simulink model "LQI_NL_simulation"  (R2024b)
settings: Solver=VariableStepAuto  StartTime=0.0  StopTime=20  RelTol=1e-3
values from neighbouring files (symbols this model uses):
  A_kf = A_ext - L_kf*C_meas    [SS_model_LQ.m]
  B_kf = [L_kf B_ext]    [SS_model_LQ.m]
  C_kf = eye(3)    [SS_model_LQ.m]
  D_kf = zeros(3,3)    [SS_model_LQ.m]
  g = 9.81    [LQI_Giuse_code.m]    (also in SS_model_LQ.m)
  G_i_num = G_i_num(2)    [SS_model_LQ.m]
  i_e = sqrt((m*g/km) * (x_e + 2*r -l)^2)    [SS_model_LQ.m]
  K_aug = lqr(A_aug, B_aug, Q_aug, R_aug)    [SS_model_LQ.m]
  Kg = 3    [LQI_Giuse_code.m]    (also in SS_model_LQ.m)
  Ki_i = Ki_p/Ti    [LQI_Giuse_code.m]    (also in SS_model_LQ.m = 1650.02619)
  km = 6.5308e-5    (= 6.5308e-05)    [LQI_Giuse_code.m]    (also in SS_model_LQ.m)
  Kp_i = 72.795273    [SS_model_LQ.m]
  l = 0.0394    [LQI_Giuse_code.m]    (also in SS_model_LQ.m)
  L = 412.5e-3    (= 0.4125)    [SS_model_LQ.m]
  m = 0.068    [LQI_Giuse_code.m]    (also in SS_model_LQ.m)
  r = 1.27e-2    (= 0.0127)    [LQI_Giuse_code.m]    (also in SS_model_LQ.m)
  R = 1    [LQI_Giuse_code.m]    (also in SS_model_LQ.m = 9.35)
  x_e = [x1_e, x2_e]    [LQI_Giuse_code.m]    (also in SS_model_LQ.m = 0.007)
undefined symbols (not defined in the file or in its folder): G_i_den
libraries: slpidlib x1
settings Model: Creator=edoardo  LastModifiedBy=edoardo

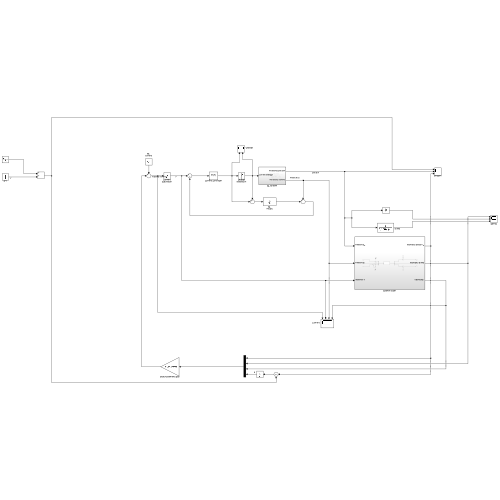
[thumbnail: Simulink's stored preview of the top-level diagram]
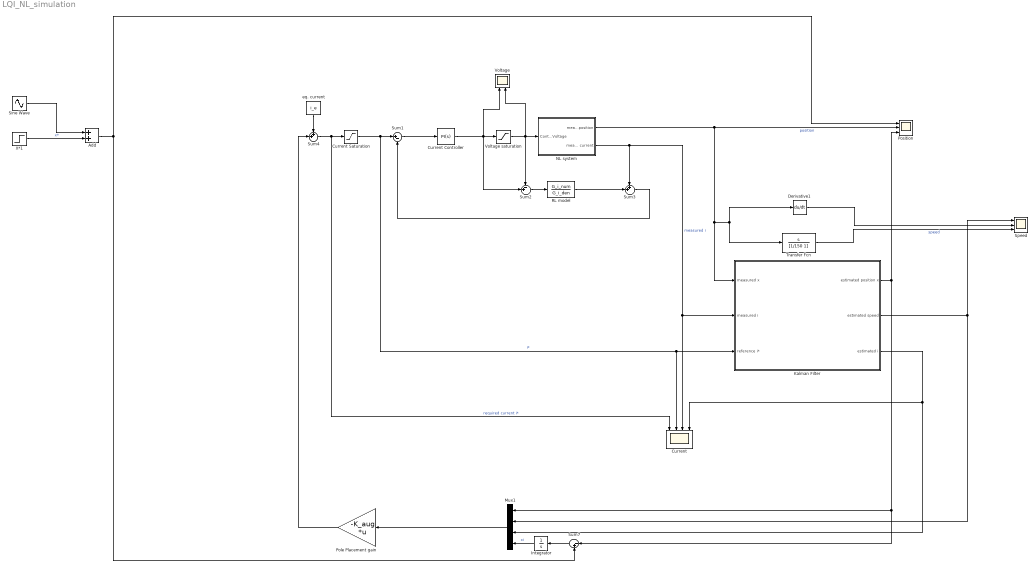
== system LQI_NL_simulation ==
  Add : Sum
  Current : Scope  NumInputPorts=4
  Current Saturation : Saturate  UpperLimit=3  LowerLimit=0
  Current Controller : slpidlib/PID Controller  Controller=PI  Form=Parallel  TimeDomain=Continuous-time  UseExternalTs=off  SampleTime=-1  IntegratorMethod=Forward Euler  FilterMethod=Forward Euler  ControllerParametersSource=internal  P=Kp_i  I=Ki_i  UseKiTs=off  D=0  UseExternalDerivativeSource=off  N=100  UseFilter=on  TunerSelectOption=Transfer Function Based (PID Tuner App)  InitialConditionSource=internal  InitialConditionForIntegrator=0  InitialConditionForFilter=0  DifferentiatorICPrevScaledInput=0  ExternalReset=none  TrackingMode=off  Kt=1  LimitOutput=off  SatLimitsSource=internal  UpperSaturationLimit=inf  LowerSaturationLimit=-inf  LinearizeAsGain=on  AntiWindupMode=none  Kb=1  LimitIntegrator=off  UpperIntegratorSaturationLimit=inf  LowerIntegratorSaturationLimit=-inf  POutMin=[]  POutMax=[]  IOutMin=[]  IOutMax=[]  DOutMin=[]  DOutMax=[]  NOutMin=[]  NOutMax=[]  SumOutMin=[]  SumOutMax=[]  SaturationOutMin=[]  SaturationOutMax=[]  PParamMin=[]  PParamMax=[]  IParamMin=[]  IParamMax=[]  DParamMin=[]  DParamMax=[]  NParamMin=[]  NParamMax=[]  KbParamMin=[]  KbParamMax=[]  KtParamMin=[]  KtParamMax=[]  KbOutMin=[]  KbOutMax=[]  KtOutMin=[]  KtOutMax=[]  IntegratorOutMin=[]  IntegratorOutMax=[]  FilterOutMin=[]  FilterOutMax=[]  SumI1OutMin=[]  SumI1OutMax=[]  SumI2OutMin=[]  SumI2OutMax=[]  SumI3OutMin=[]  SumI3OutMax=[]  SumI4OutMin=[]  SumI4OutMax=[]  SumDOutMin=[]  SumDOutMax=[]  DifferentiatorOutMin=[]  DifferentiatorOutMax=[]  FilterDiffOutCoefMin=[]  FilterDiffOutCoefMax=[]  ReciprocalOutMin=[]  ReciprocalOutMax=[]  SumDenOutMin=[]  SumDenOutMax=[]  SumNumOutMin=[]  SumNumOutMax=[]  DivideOutMin=[]  DivideOutMax=[]  UdiffTsProdOutMin=[]  UdiffTsProdOutMax=[]  NTsProdOutMin=[]  NTsProdOutMax=[]  UintegralTsProdOutMin=[]  UintegralTsProdOutMax=[]  UngainTsProdOutMin=[]  UngainTsProdOutMax=[]  ClampingZeroOutDataTypeStr=Inherit: Inherit via back propagation  ClampingZeroOutMin=[]  ClampingZeroOutMax=[]  FilterDenConstantOutDataTypeStr=Inherit: Inherit via back propagation  FilterDenConstantOutMin=[]  FilterDenConstantOutMax=[]  PCopyOutDataTypeStr=Inherit: Inherit via back propagation  PCopyOutMin=[]  PCopyOutMax=[]  NCopyOutDataTypeStr=Inherit: Inherit via back propagation  NCopyOutMin=[]  NCopyOutMax=[]  IntegratorContinuousStateAttributes=''  IntegratorStateMustResolveToSignalObject=off  IntegratorRTWStateStorageClass=Auto  FilterContinuousStateAttributes=''  FilterStateMustResolveToSignalObject=off  FilterRTWStateStorageClass=Auto  ParallelPVariant=InternalParameters  IdealPVariant=Disabled  IVariant=InternalParameters  DVariant=Disabled  IntegratorVariant=Continuous  SatVariant=Disabled  AWVariant=Passthrough  PCopyVariant=Disabled  TRVariant=Disabled  FdbkBlocksVariant=Forward  IdealPFdbkVariant=Disabled  SatFdbkVariant=Disabled  DerivativeFilterVariant=Disabled  NVariant=Disabled  NCopyVariant=Disabled_SignalSpec  FilterICVariant=Disabled  IntegratorICVariant=InternalICs  ExternalResetVariant=Disabled  TRSumVariant=Passthrough  SumFdbkVariant=Disabled  SumVariant=Sum_PI  TsampFilterVariant=InternalTs  TsampNgainVariant=Passthrough  TsampIntegralVariant=Disabled_SignalSpec  ExternalSaturationOutDataTypeStr=Inherit: Same as second input  DerivativeSourceVariant=Disabled  PreIntVariant=InternalPreInt
  Derivative1 : Derivative
  Integrator : Integrator
  Kalman Filter : Subsystem
  Mux1 : Mux
  NL system : Subsystem
  Pole Placement gain : Gain  Gain=-K_aug  Multiplication=Matrix(K*u) (u vector)
  Position : Scope  NumInputPorts=3
  RL model : TransferFcn  Numerator=G_i_num  Denominator=G_i_den
  Sine Wave : Sin  Amplitude=0  SampleTime=0
  Speed : Scope  NumInputPorts=3
  Sum1 : Sum  Inputs=|+-
  Sum2 : Sum  Inputs=-+|
  Sum3 : Sum  Inputs=++|
  Sum4 : Sum  Inputs=++|
  Sum7 : Sum  Inputs=|-+
  Transfer Fcn : TransferFcn  Numerator=[1 0]  Denominator=[1/150 1]
  Voltage : Scope  NumInputPorts=2
  Voltage saturation : Saturate  UpperLimit=8  LowerLimit=-8
  X*1 : Step  After=x_e  SampleTime=0
  eq. current : Constant  Value=i_e
  wires:
  Current Controller/1 -> Voltage/1, Sum2/2, Voltage saturation/1
  RL model/1 -> Sum3/2
  Sum3/1 -> Sum1/2
  Sum2/1 -> RL model/1
  Voltage saturation/1 -> NL system/1(Control Voltage), Voltage/2, Sum2/1
  Sum1/1 -> Current Controller/1
  Current Saturation/1 -> Kalman Filter/3(reference i*), Current/2, Sum1/1  "i*"
  Transfer Fcn/1 -> Speed/3  "speed"
  Mux1/1 -> Pole Placement gain/1
  eq. current/1 -> Sum4/1
  Derivative1/1 -> Speed/2
  NL system/2(measured current) -> Kalman Filter/2(measured i), Current/3, Sum3/1  "measured i"
  Sum4/1 -> Current/1, Current Saturation/1  "required current i*"
  Kalman Filter/1(estimated position x) -> Position/3, Mux1/1, Sum7/1
  Kalman Filter/3(estimated i) -> Current/4, Mux1/3
  Kalman Filter/2(estimated speed) -> Speed/1, Mux1/2
  NL system/1(measured position) -> Kalman Filter/1(measured x), Derivative1/1, Transfer Fcn/1, Position/2  "position"
  Pole Placement gain/1 -> Sum4/2
  Sum7/1 -> Integrator/1
  Integrator/1 -> Mux1/4  "xi"
  Add/1 -> Position/1, Sum7/2
  Sine Wave/1 -> Add/1
  X*1/1 -> Add/2  "x*"

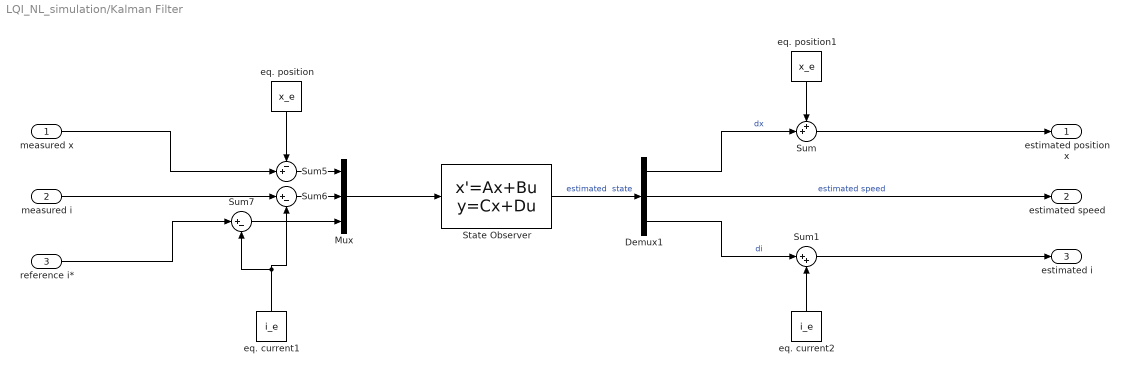
== system LQI_NL_simulation/Kalman Filter ==
  measured x : Inport
  measured i : Inport  Port=2
  reference i* : Inport  Port=3
  Demux1 : Demux  Outputs=3
  Mux : Mux  Inputs=3
  State Observer : StateSpace  A=A_kf  B=B_kf  C=C_kf  D=D_kf  InitialCondition=0
  Sum : Sum  Inputs=++|
  Sum1 : Sum  Inputs=|++
  Sum5 : Sum  Inputs=-+|
  Sum6 : Sum  Inputs=|+-
  Sum7 : Sum  Inputs=|+-
  eq. current1 : Constant  Value=i_e
  eq. current2 : Constant  Value=i_e
  eq. position : Constant  Value=x_e
  eq. position1 : Constant  Value=x_e
  estimated position x : Outport
  estimated speed : Outport  Port=2
  estimated i : Outport  Port=3
  wires:
  eq. position/1 -> Sum5/1
  State Observer/1 -> Demux1/1  "estimated  state"
  Sum7/1 -> Mux/3
  Sum6/1 -> Mux/2
  Mux/1 -> State Observer/1
  Sum5/1 -> Mux/1
  measured x/1 -> Sum5/2
  measured i/1 -> Sum6/1
  reference i*/1 -> Sum7/1
  Demux1/1 -> Sum/2  "dx"
  Sum/1 -> estimated position x/1
  eq. position1/1 -> Sum/1
  eq. current2/1 -> Sum1/2
  Sum1/1 -> estimated i/1
  Demux1/2 -> estimated speed/1  "estimated speed"
  Demux1/3 -> Sum1/1  "di"
  eq. current1/1 -> Sum7/2, Sum6/2

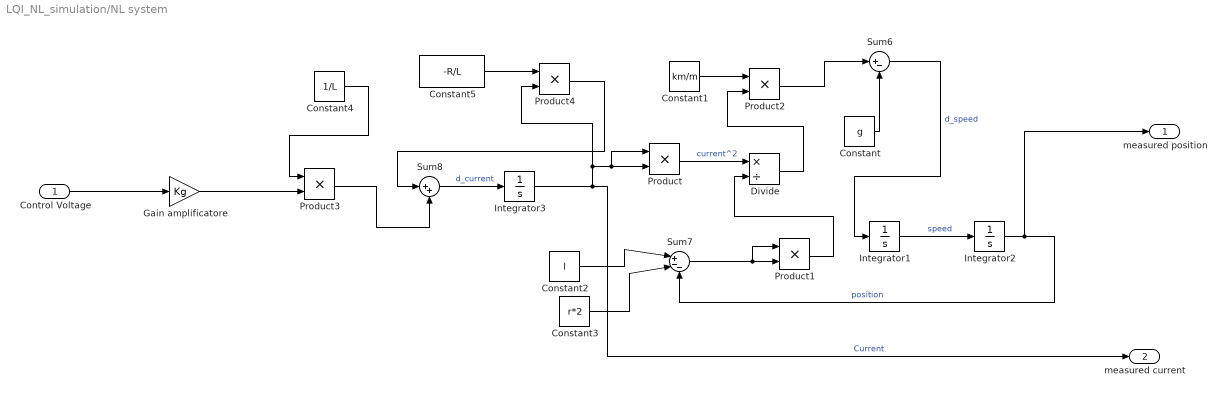
== system LQI_NL_simulation/NL system ==
  Control Voltage : Inport
  Constant : Constant  Value=g
  Constant1 : Constant  Value=km/m
  Constant2 : Constant  Value=l
  Constant3 : Constant  Value=r*2
  Constant4 : Constant  Value=1/L
  Constant5 : Constant  Value=-R/L
  Divide : Product  Inputs=*/
  Gain amplificatore : Gain  Gain=Kg
  Integrator1 : Integrator
  Integrator2 : Integrator  LimitOutput=on  UpperSaturationLimit=0.014  LowerSaturationLimit=0
  Integrator3 : Integrator
  Product{,1..4} (5 alike) : Product
  Sum6 : Sum  Inputs=|+-
  Sum7 : Sum  Inputs=|+--
  Sum8 : Sum  Inputs=|++
  measured position : Outport
  measured current : Outport  Port=2
  wires:
  Divide/1 -> Product2/2
  Constant3/1 -> Sum7/2
  Constant/1 -> Sum6/2
  Sum6/1 -> Integrator1/1  "d_speed"
  Constant1/1 -> Product2/1
  Product/1 -> Divide/1  "current^2"
  Control Voltage/1 -> Gain amplificatore/1
  Product4/1 -> Sum8/1
  Product1/1 -> Divide/2
  Sum7/1 -> Product1/2, Product1/1
  Product3/1 -> Sum8/2
  Integrator1/1 -> Integrator2/1  "speed"
  Constant4/1 -> Product3/1
  Product2/1 -> Sum6/1
  Constant5/1 -> Product4/1
  Sum8/1 -> Integrator3/1  "d_current"
  Integrator2/1 -> measured position/1, Sum7/3  "position"
  Constant2/1 -> Sum7/1
  Integrator3/1 -> measured current/1, Product4/2, Product/2, Product/1  "Current"
  Gain amplificatore/1 -> Product3/2
